simulink model "Bdot"  (R2023b)
settings: Solver=VariableStepAuto  StartTime=0.0  StopTime=10.0  RelTol=1e-3
libraries: aerolibutil x1
settings Model: Creator=Adin Sacho-Tanzer  LastModifiedBy=Adin Sacho-Tanzer

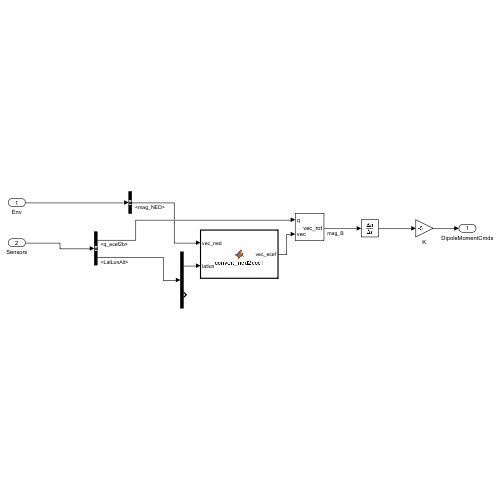
[thumbnail: Simulink's stored preview of the top-level diagram]
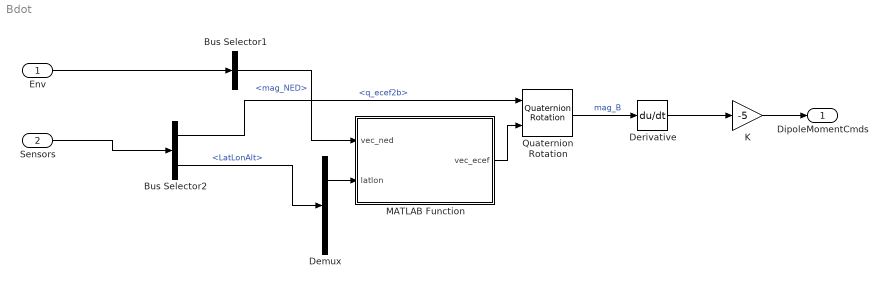
== system Bdot ==
  Env : Inport
  Sensors : Inport  Port=2
  Bus Selector1 : BusSelector  OutputSignals=mag_NED
  Bus Selector2 : BusSelector  OutputSignals=q_ecef2b,LatLonAlt
  Demux : Demux  Outputs=[2 1]
  Derivative : Derivative
  K : Gain  Gain=-5
  MATLAB Function : MATLAB Function  TreatAsAtomicUnit=on
  Quaternion Rotation : aerolibutil/Quaternion Rotation
  DipoleMomentCmds : Outport
  wires:
  MATLAB Function/1(vec_ecef) -> Quaternion Rotation/2
  Bus Selector2/1 -> Quaternion Rotation/1  "<q_ecef2b>"
  Demux/1 -> MATLAB Function/2(latlon)
  Sensors/1 -> Bus Selector2/1
  Bus Selector1/1 -> MATLAB Function/1(vec_ned)  "<mag_NED>"
  Env/1 -> Bus Selector1/1
  Bus Selector2/2 -> Demux/1  "<LatLonAlt>"
  Quaternion Rotation/1 -> Derivative/1  "mag_B"
  Derivative/1 -> K/1
  K/1 -> DipoleMomentCmds/1

== matlab function Bdot/MATLAB Function ==
  data: vec_ned input; vec_ecef output double size=[3 1]; latlon input
function vec_ecef = convert_ned2ecef(vec_ned, latlon)

vec_ecef = zeros(3,1);

uN = vec_ned(1);
vE = vec_ned(2);
wD = vec_ned(3);

lat = deg2rad(latlon(1));
lon = deg2rad(latlon(2));

sLat = sin(lat);
cLat = cos(lat);
sLon = sin(lon);
cLon = cos(lon);

vec_ecef(1) = -sLat*cLon*uN - sLon*vE - cLat*cLon*wD;
vec_ecef(2) = -sLat*sLon*uN + cLon*vE - cLat*sLon*wD;
vec_ecef(3) =  cLat*uN              - sLat*wD;

end
